simulink model "cubesat_alg_dev_env_v2_bugged"  (R2024a)
settings: Solver=FixedStepAuto  StartTime=0.0  StopTime=7200  FixedStep=0.01  MaxStep=1  MinStep=0.01  RelTol=1e-3
model workspace (MAT data in the model file):
  visSampleTime = 3
undefined symbols (not defined in the file or in its folder): WMM2020
libraries: aerolibutil x9, matrix_library x6, vrlib x4, sharedtransform x2, aerolibgravity2 x2, dspinverses x1, sharedutil x1, simulink_extras x1
(part 2 of 2)

== matlab function cubesat_alg_dev_env_v2_bugged/attitude_determination_and_vehicle_est/MEKF ==
  data: P input; P output; q_n2m input; beta input; q_n2m output; beta output; omega input; ref_ss input; mes_ss input; use_sun_sensor input; ref_mag input; mes_mag input; use_magnometer input; ref_aam input; mes_aam input; use_ang_acc_magentorquer input; use_ang_vel input; mes_var_ss input; mes_var_mg input; mes_var_aam input; dt input; hat_omega output size=[3,1]; use_steve_mode input; steve_ref input; steve_mes input
function [P, q_n2m,beta,hat_omega] = MEKF(P,q_n2m,beta,omega, ref_ss, mes_ss, use_sun_sensor, ref_mag, mes_mag, ...
                                            use_magnometer, ref_aam, mes_aam, use_ang_acc_magentorquer, use_ang_vel, ...
                                            mes_var_ss, mes_var_mg, mes_var_aam, dt, use_steve_mode, steve_ref, steve_mes)

    [P, q_n2m,beta,hat_omega] = fullMEKF(P,q_n2m,beta,omega, ref_ss, mes_ss, use_sun_sensor, ref_mag, mes_mag, ...
                                                use_magnometer, ref_aam, mes_aam, use_ang_acc_magentorquer, use_ang_vel, ...
                                                mes_var_ss, mes_var_mg, mes_var_aam, dt, use_steve_mode, steve_ref, steve_mes);
    
end


%     delta_x = zeros(6,1);
% 
%     G = [-eye(3), zeros(3);
%     zeros(3), eye(3)];
% 
%     Q = [mes_var_ss^2*eye(3), zeros(3);
%     zeros(3), mes_var_mg^2*eye(3)];
% 
%     %sun sensor
%     if use_sun_sensor
%     [q_n2m,P,delta_x] = mekf(mes_ss,ref_ss,P,mes_var_ss,q_n2m,delta_x);
%     end
% 
%     %magnometer
%     if use_magnometer
%     [q_n2m,P,delta_x] = mekf(mes_mag,ref_mag,P,mes_var_mg,q_n2m,delta_x);
%     end
% 
%     %steve mode
%     if use_steve_mode 
%         steve_mes_reshape = reshape(steve_mes,[1 3]);
%         steve_ref_reshape = reshape(steve_ref,[1 3]);
%         [q_n2m,P,delta_x] = mekf(steve_mes_reshape,steve_ref_reshape,P,0.1,q_n2m,delta_x);
%     end
% 
%     %angular velocity with accelerometer
%     %if use_ang_acc_magentorquer
%     %[q_n2m,P,delta_x] = mekf(mes_aam,ref_aam,P,mes_var_aam,q_n2m,delta_x);
%     %end
% 
% 
%     x_extra = [0 ; delta_x(1:3)]';
% 
%     q_n2m = q_n2m + (0.5*quatmultiply(q_n2m,x_extra));
%     q_n2m = q_n2m/norm(q_n2m);
% 
%     hat_omega = zeros(3,1);
%     if use_ang_vel
%         %beta = beta + delta_x(4:6);
%         hat_omega(1) = omega(1) - beta(1);
%         hat_omega(2) = omega(2) - beta(2);
%         hat_omega(3) = omega(3) - beta(3);
%     end
% 
%     x_extra = [0; hat_omega]';
%     dot_q_n2m = 0.5*quatmultiply(q_n2m,x_extra);
% 
%     q_n2m = q_n2m + dot_q_n2m*dt;
%     q_n2m = q_n2m/norm(q_n2m);
% 
%     w = [ 0  -hat_omega(3),  hat_omega(2);
%           hat_omega(3),    0, -hat_omega(1);
%          -hat_omega(2),  hat_omega(1),    0];
% 
%     F = [-w, eye(3);
%         zeros(3), zeros(3)];
% 
%     dot_P = F*P + P*F'+G*Q*G';
% 
%     P = P + dot_P*dt;
% 
% end
% 
% 
% function [q_n2m,P,delta_x] = mekf(b,r,P,R,q_n2m, delta_x)
% 
%     b_est = quatrotate(q_n2m,r);
%     b01 = b_est(1);
%     b02 = b_est(2);
%     b03 = b_est(3);
% 
% 
%     H = [   0  -b03,  b02,  0,  0,  0;
%           b03,    0, -b01,  0,  0,  0;
%          -b02,  b01,    0,  0,  0,  0];
% 
%     K = P*transpose(H)/(H*P*transpose(H)+R^2*eye(3));
% 
%     epsilon = (b - quatrotate(q_n2m,r));
% 
%     delta_x = delta_x + K*(epsilon'-H*delta_x);
% 
%     P = (eye(6) - K*H)*P;
% 
% end
% 
% function v = quatrotate(q,v)
% q0 = q(1);
% q1 = q(2);
% q2 = q(3);
% q3 = q(4);
% 
% M = zeros(3);
% 
% M(1,1) = 1 - 2*q2^2 - 2*q3^2;
% M(1,2) = 2*(q1*q2 + q0*q3);
% M(1,3) = 2*(q1*q3-q0*q2);
% M(2,1) = 2*(q1*q2-q0*q3);
% M(2,2) = 1 - 2*q1^2 - 2*q3^2;
% M(2,3) = 2*(q2*q3+q0*q1);
% M(3,1) = 2*(q1*q3+q0*q2);
% M(3,2) = 2*(q2*q3-q0*q1);
% M(3,3) = 1 - 2*q2^2 - 2*q3^2;
% 
% v = (M*(v'))';
% end

== matlab function cubesat_alg_dev_env_v2_bugged/sens_modelling/MATLAB Function4 ==
  data: u input; y output
function y = signal_cleanup(u)
y = [0,0,0];

if u(1) == 0
    y(1) = -u(2);
else
    y(1) = u(1);
end

if u(3) == 0
    y(2) = -u(4);
else
    y(2) = u(3);
end

if u(5) == 0
    y(3) = -u(6);
else
    y(3) = u(5);
end


end

== matlab function cubesat_alg_dev_env_v2_bugged/env_modelling/MATLAB Function ==
  data: pos_gci input; torque_body output; iner_tensor input
function torque_body  = grav_grad_torque(pos_gci, iner_tensor)
    % mass of earth, grav constant
    m_e = 5.97219e24;
    G = 6.67430e-11;

    % grav param
    u = G*m_e;

    radius = norm(pos_gci);
    nadir_vec = -normalize(pos_gci);
    torque_body = cross(3*u/radius^3*nadir_vec, ...
        iner_tensor*nadir_vec);

== matlab function cubesat_alg_dev_env_v2_bugged/SSD Memory Access/Earth Presession ==
  data: u input; y output
function y = fcn(u)

y = u;

== matlab function cubesat_alg_dev_env_v2_bugged/datetime_modelling_and_ref_frames/MATLAB Function1 ==
  data: datetime input; dyear output
function dyear = dyear_from_datetime(datetime)

    % the datetime format is provided as a 6 value array
    % year, month, day, hour, minute, second

    % sequentially builds the decimal year

    % potentially we may want to use /61 for leap second days but this is
    % likely fine as our simulation just needs to perform regular datetime
    % updates for simple testing

    tot_mins = datetime(5) + datetime(6) / 60;
    tot_hours = datetime(4) + tot_mins / 60;
    tot_days = datetime(3) + tot_hours / 24;
    tot_months = datetime(2) + tot_days / (275/9); % average days in month across year
    tot_years = datetime(1) + tot_months / 12;

    dyear = tot_years;

== matlab function cubesat_alg_dev_env_v2_bugged/onboad_env_modelling/MATLAB Function6 ==
  data: u input; y output
function y = noise_sim(u)

y = u;
